simulink model "vardownsampler"  (Simulink 7.3)
settings: Solver=VariableStepDiscrete  StartTime=0.0  StopTime=simTime*SampleTime  RelTol=1e-3
PreLoadFcn:
  | setup_vardownsampler
InitFcn:
  | setup_vardownsampler
values from neighbouring files (symbols this model uses):
  accumOutShift = [1 4 3 2 4]    [setup_vardownsampler.m]    (also in setup_vardownsamplerL8.m = [3 3 2 2 2])
  accumOutWidth = dataWidth + ceil(log2(Rmax))+0    [setup_vardownsampler.m]    (also in setup_vardownsamplerL8.m)
  adderOutShift = 4*ones(1,numRates)    [setup_vardownsampler.m]    (also in setup_vardownsamplerL8.m = 3*ones(1,numRates))
  adderOutWidth = dataWidth + coeffWidth + ceil(log2(L))    [setup_vardownsampler.m]    (also in setup_vardownsamplerL8.m)
  addrWidth = max(1,ceil(log2(Rmax)))    [setup_vardownsampler.m]    (also in setup_vardownsamplerL8.m)
  ChanCount = 16    [setup_vardownsampler.m]    (also in setup_vardownsamplerL8.m = 1)
  ChanCycleCount = ceil(ChanCount/ChanWireCount)    [setup_vardownsampler.m]    (also in setup_vardownsamplerL8.m)
  ChanWireCount = ceil(ChanCount/Period)    [setup_vardownsampler.m]    (also in setup_vardownsamplerL8.m)
  coeffWidth = 16    [setup_vardownsampler.m]    (also in setup_vardownsamplerL8.m)
  dataWidth = 16    [setup_vardownsampler.m]    (also in setup_vardownsamplerL8.m)
  FirAddr = AccumOutScale + 1    (= 4)    [setup_vardownsampler.m]    (also in setup_vardownsamplerL8.m)
  hmatrix = zeros(2*Rmax, L)    [setup_vardownsampler.m]    (also in setup_vardownsamplerL8.m)
  memAddrWidth = max(1,ceil(log2(Nmax)))    [setup_vardownsampler.m]    (also in setup_vardownsamplerL8.m)
  Nmax = Period*Rmax    [setup_vardownsampler.m]    (also in setup_vardownsamplerL8.m)
  Period = floor(ClockRate / SampleRate)    [setup_vardownsampler.m]    (also in setup_vardownsamplerL8.m)
  R = [1 2 5 8 2]    [setup_vardownsampler.m]    (also in setup_vardownsamplerL8.m = [4 5 7 8 9])
  RateWidth = ceil(log2(Rmax))+1    [setup_vardownsampler.m]    (also in setup_vardownsamplerL8.m)
  resetCntWidth = max(1,ceil(log2(Nmax)))    [setup_vardownsampler.m]    (also in setup_vardownsamplerL8.m)
  Rmax = 16    [setup_vardownsampler.m]    (also in setup_vardownsamplerL8.m = 20)
  SampleTime = 1    [setup_vardownsampler.m]    (also in setup_vardownsamplerL8.m)
undefined symbols (not defined in the file or in its folder): AdvDSPBChannelOutDisplay, AdvDSPBDMemDisplay, bank1, bank2, c4, c5, c6, c7, c8, c9, dpoly, dspba_ChannelInVis, dspba_ChannelOutVis, dspba_internal_get_channel_ports, evalAionMaskParam, hmatrix0, hmatrix1, hmatrix2, hmatrix3, latency, primtype, UseDontCare, value
libraries: DSPBAPrim x314, DSPBAModelBus x24, simulink x12, DSPBABase x6
(part 3 of 4)

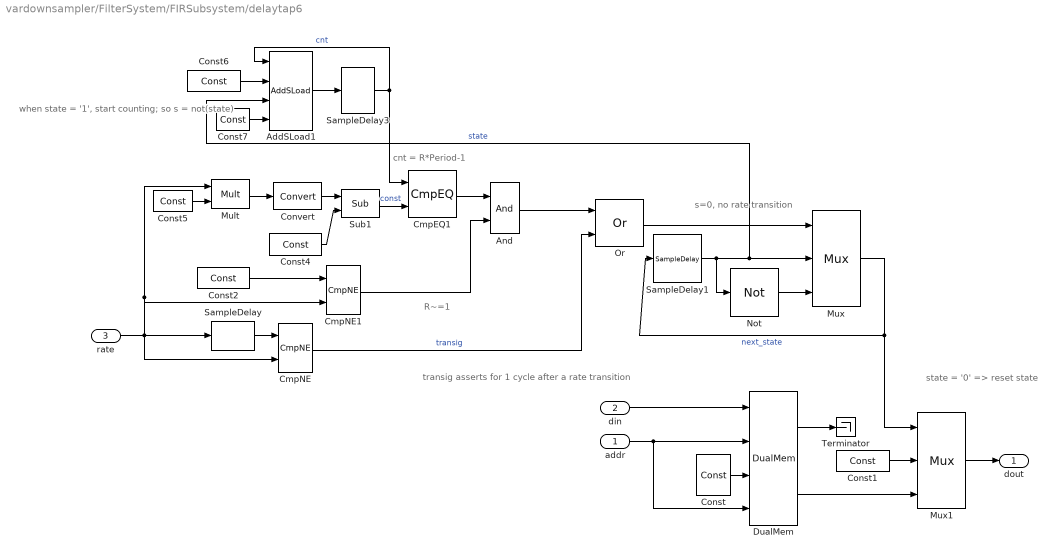
== system vardownsampler/FilterSystem/FIRSubsystem/delaytap6 ==
  note: s=0, no rate transition
  note: transig asserts for 1 cycle after a rate transition
  note: cnt = R*Period-1
  note: when state = '1', start counting;
      | so s = not(state)
  note: state = '0' => reset state
  note: R~=1
  addr : Inport
  din : Inport  Port=2
  rate : Inport  Port=3
  AddSLoad1 : DSPBAPrim/AddSLoad  primtype=addsload  nInputs=4  nOutputs=1  omode=Specify via dialog  otype=uint(resetCntWidth)  scale=1  rndmethod=Unbiased  factor=1  satmethod=Symmetric  shift_vec=[0 1 2 -1]  value=0  inPortNames=['+'; '+'; 's'; 'v']  outPortNames=[' ']  image=dspba_prim.jpg  text=fprintf('+');  style=Optimised  visibilities=8  version=20090407
  And : DSPBAPrim/And  primtype=and  nInputs=2  nOutputs=1  omode=Inherit via internal rule  otype=sfix(16)  scale=2^-15  rndmethod=Unbiased  factor=1  satmethod=Symmetric  shift_vec=[0 1 2 -1]  value=0  inPortNames=[' '; ' '; ' '; ' '; ' '; ' '; ' '; ' '; ' '; ' '; ' '; ' '; ' '; ' '; ' '; ' '; ]  outPortNames=[' ']  image=dspba_prim.jpg  text=fprintf('&');  style=Optimised  visibilities=8+2  version=20090407
  CmpEQ1 : DSPBAPrim/CmpEQ  primtype=cmpeq  nInputs=2  nOutputs=1  omode=boolean  otype=sfix(16)  scale=2^-15  rndmethod=Unbiased  factor=1  satmethod=Symmetric  shift_vec=[0 1 2 -1]  value=0  inPortNames=[' '; ' ';]  outPortNames=[' ']  image=dspba_prim.jpg  text=fprintf('==');  style=Optimised  visibilities=0  version=20090407
  CmpNE : DSPBAPrim/CmpNE  primtype=cmpne  nInputs=2  nOutputs=1  omode=boolean  otype=sfix(16)  scale=2^-15  rndmethod=Unbiased  factor=1  satmethod=Symmetric  shift_vec=[0 1 2 -1]  value=0  inPortNames=[' '; ' ';]  outPortNames=[' ']  image=dspba_prim.jpg  text=fprintf('~=');  style=Optimised  visibilities=0  version=20090407
  CmpNE1 : DSPBAPrim/CmpNE  primtype=cmpne  nInputs=2  nOutputs=1  omode=boolean  otype=sfix(16)  scale=2^-15  rndmethod=Unbiased  factor=1  satmethod=Symmetric  shift_vec=[0 1 2 -1]  value=0  inPortNames=[' '; ' ';]  outPortNames=[' ']  image=dspba_prim.jpg  text=fprintf('~=');  style=Optimised  visibilities=0  version=20090407
  Const : DSPBAPrim/Const  primtype=const  nInputs=0  nOutputs=1  omode=Inherit via internal rule  otype=sfix(16)  scale=2^-15  rndmethod=Unbiased  factor=1  satmethod=Symmetric  shift_vec=[0 1 2 -1]  value=1  inPortNames=['+'; '+';]  outPortNames=[' ']  image=dspba_prim.jpg  text=fprintf('%s', num2str(value));  style=Optimised  visibilities=8 + 1024  version=20090407
  Const1 : DSPBAPrim/Const  primtype=const  nInputs=0  nOutputs=1  omode=Specify via dialog  otype=sfix(dataWidth)  scale=2^(-dataWidth+1)  rndmethod=Unbiased  factor=1  satmethod=Symmetric  shift_vec=[0 1 2 -1]  value=0  inPortNames=['+'; '+';]  outPortNames=[' ']  image=dspba_prim.jpg  text=fprintf('%s', num2str(value));  style=Optimised  visibilities=8 + 1024  version=20090407
  Const2 : DSPBAPrim/Const  primtype=const  nInputs=0  nOutputs=1  omode=Specify via dialog  otype=uint(RateWidth)  scale=1  rndmethod=Unbiased  factor=1  satmethod=Symmetric  shift_vec=[0 1 2 -1]  value=1  inPortNames=['+'; '+';]  outPortNames=[' ']  image=dspba_prim.jpg  text=fprintf('%s', num2str(value));  style=Optimised  visibilities=8 + 1024  version=20090407
  Const4 : DSPBAPrim/Const  primtype=const  nInputs=0  nOutputs=1  omode=Specify via dialog  otype=uint(resetCntWidth)  scale=1  rndmethod=Unbiased  factor=1  satmethod=Symmetric  shift_vec=[0 1 2 -1]  value=1  inPortNames=['+'; '+';]  outPortNames=[' ']  image=dspba_prim.jpg  text=fprintf('%s', num2str(value));  style=Optimised  visibilities=8 + 1024  version=20090407
  Const5 : DSPBAPrim/Const  primtype=const  nInputs=0  nOutputs=1  omode=Specify via dialog  otype=uint(resetCntWidth)  scale=1  rndmethod=Unbiased  factor=1  satmethod=Symmetric  shift_vec=[0 1 2 -1]  value=Period  inPortNames=['+'; '+';]  outPortNames=[' ']  image=dspba_prim.jpg  text=fprintf('%s', num2str(value));  style=Optimised  visibilities=8 + 1024  version=20090407
  Const6 : DSPBAPrim/Const  primtype=const  nInputs=0  nOutputs=1  omode=Specify via dialog  otype=uint(resetCntWidth)  scale=1  rndmethod=Unbiased  factor=1  satmethod=Symmetric  shift_vec=[0 1 2 -1]  value=1  inPortNames=['+'; '+';]  outPortNames=[' ']  image=dspba_prim.jpg  text=fprintf('%s', num2str(value));  style=Optimised  visibilities=8 + 1024  version=20090407
  Const7 : DSPBAPrim/Const  primtype=const  nInputs=0  nOutputs=1  omode=Specify via dialog  otype=uint(resetCntWidth)  scale=1  rndmethod=Unbiased  factor=1  satmethod=Symmetric  shift_vec=[0 1 2 -1]  value=0  inPortNames=['+'; '+';]  outPortNames=[' ']  image=dspba_prim.jpg  text=fprintf('%s', num2str(value));  style=Optimised  visibilities=8 + 1024  version=20090407
  Convert : DSPBAPrim/Convert  primtype=convert  nInputs=1  nOutputs=1  omode=Specify via dialog  otype=uint(resetCntWidth)  scale=1  rndmethod=Truncate  factor=1  satmethod=None  shift_vec=[0 1 2 -1]  value=round([0:255]/17)  inPortNames=[' '; ' ';]  outPortNames=[' '; 'c']  image=dspba_prim.jpg  text=fprintf('convert');  style=Optimised  visibilities=8+64+256  clipdetect=off  version=20090611
  DualMem : DSPBAPrim/DualMem  primtype=dualmem  nInputs=4  nOutputs=2  omode=Inherit via internal rule  otype=sfix(16)  scale=2^-15  rndmethod=Unbiased  factor=1  satmethod=Symmetric  shift_vec=[0 1 2 -1]  value=[zeros(Nmax, 1)]  inPortNames=['d'; 'a'; 'w'; 'a']  outPortNames=['q1'; 'q2']  image=dspba_prim.jpg  text=fprintf('dmem%s',AdvDSPBDMemDisplay(UseDontCare));  style=Optimised  visibilities=8 + 1024  UseDontCare=off  version=20090407
  Mult : DSPBAPrim/Mult  primtype=mult  nInputs=2  nOutputs=1  omode=Inherit via internal rule  otype=sfix(16)  scale=2^-15  rndmethod=Unbiased  factor=1  satmethod=Symmetric  shift_vec=[0 1 2 -1]  value=0  inPortNames=[' '; ' ';]  outPortNames=[' ']  image=dspba_prim.jpg  text=fprintf('X');  style=Optimised  visibilities=8  version=20090407
  Mux : DSPBAPrim/Mux  primtype=mux  nInputs=evalAionMaskParam(gcb,'value',1)+1  nOutputs=1  omode=Inherit via internal rule  otype=sfix(16)  scale=2^-15  rndmethod=Unbiased  factor=1  satmethod=Symmetric  shift_vec=[0 1 2 -1]  value=2  inPortNames=['s'; 'd0'; 'd1'; 'd2'; 'd3'; 'd4'; 'd5'; 'd6'; 'd7'; 'd8'; 'd9';]  outPortNames=[' ']  image=dspba_prim.jpg  text=fprintf('%s', primtype);  style=Optimised  visibilities=1032  version=20090623
  Mux1 : DSPBAPrim/Mux  primtype=mux  nInputs=evalAionMaskParam(gcb,'value',1)+1  nOutputs=1  omode=Inherit via internal rule  otype=sfix(16)  scale=2^-15  rndmethod=Unbiased  factor=1  satmethod=Symmetric  shift_vec=[0 1 2 -1]  value=2  inPortNames=['s'; 'd0'; 'd1'; 'd2'; 'd3'; 'd4'; 'd5'; 'd6'; 'd7'; 'd8'; 'd9';]  outPortNames=[' ']  image=dspba_prim.jpg  text=fprintf('%s', primtype);  style=Optimised  visibilities=1032  version=20090623
  Not : DSPBAPrim/Not  primtype=not  nInputs=1  nOutputs=1  omode=Inherit via internal rule  otype=sfix(16)  scale=2^-15  rndmethod=Unbiased  factor=1  satmethod=Symmetric  shift_vec=[0 1 2 -1]  value=0  inPortNames=[' '; ' ';]  outPortNames=[' ']  image=dspba_prim.jpg  text=fprintf('~');  style=Optimised  visibilities=8  version=20090407
  Or : DSPBAPrim/Or  primtype=or  nInputs=2  nOutputs=1  omode=Inherit via internal rule  otype=sfix(16)  scale=2^-15  rndmethod=Unbiased  factor=1  satmethod=Symmetric  shift_vec=[0 1 2 -1]  value=0  inPortNames=[' '; ' '; ' '; ' '; ' '; ' '; ' '; ' '; ' '; ' '; ' '; ' '; ' '; ' '; ' '; ' '; ]  outPortNames=[' ']  image=dspba_prim.jpg  text=fprintf('|');  style=Optimised  visibilities=8+2  version=20090407
  SampleDelay : DSPBAPrim/SampleDelay  primtype=sampdelay  nInputs=1  nOutputs=1  omode=Inherit via internal rule  otype=sfix(16)  scale=2^-15  rndmethod=Unbiased  factor=1  satmethod=Symmetric  shift_vec=[0 1 2 -1]  value=1  inPortNames=[' '; ' ';]  outPortNames=[' ']  image=dspba_prim.jpg  text=dpoly(1, eye(1,value+1), 'z')  style=Optimised  visibilities=8 + 1024  version=20090407
  SampleDelay1 : DSPBAPrim/SampleDelay  primtype=sampdelay  nInputs=1  nOutputs=1  omode=boolean  otype=sfix(16)  scale=2^-15  rndmethod=Unbiased  factor=1  satmethod=Symmetric  shift_vec=[0 1 2 -1]  value=1  inPortNames=[' '; ' ';]  outPortNames=[' ']  image=dspba_prim.jpg  text=dpoly(1, eye(1,value+1), 'z')  style=Optimised  visibilities=8 + 1024  version=20090407
  SampleDelay3 : DSPBAPrim/SampleDelay  primtype=sampdelay  nInputs=1  nOutputs=1  omode=Inherit via internal rule  otype=uint(memAddrWidth)  scale=1  rndmethod=Unbiased  factor=1  satmethod=Symmetric  shift_vec=[0 1 2 -1]  value=1  inPortNames=[' '; ' ';]  outPortNames=[' ']  image=dspba_prim.jpg  text=dpoly(1, eye(1,value+1), 'z')  style=Optimised  visibilities=8 + 1024  version=20090407
  Sub1 : DSPBAPrim/Sub  primtype=sub  nInputs=2  nOutputs=1  omode=Specify via dialog  otype=uint(memAddrWidth)  scale=1  rndmethod=Unbiased  factor=1  satmethod=Symmetric  shift_vec=[0 1 2 -1]  value=0  inPortNames=['+'; '-';]  outPortNames=[' ']  image=dspba_prim.jpg  text=fprintf('-');  style=Optimised  visibilities=8  version=20090407
  Terminator : Terminator
  dout : Outport  OutDataType=fixdt(1, 16)  OutScaling=2^0
  wires:
  Mux/1 -> SampleDelay1/1, Mux1/1  "next_state"
  SampleDelay/1 -> CmpNE/1
  rate/1 -> SampleDelay/1, CmpNE/2, Mult/1, CmpNE1/2
  CmpNE/1 -> Or/2  "transig"
  Const4/1 -> Sub1/2
  Mult/1 -> Convert/1
  Sub1/1 -> CmpEQ1/2  "const"
  Const5/1 -> Mult/2
  Convert/1 -> Sub1/1
  Const6/1 -> AddSLoad1/2
  AddSLoad1/1 -> SampleDelay3/1
  SampleDelay3/1 -> AddSLoad1/1, CmpEQ1/1  "cnt"
  Const7/1 -> AddSLoad1/4
  Or/1 -> Mux/1
  SampleDelay1/1 -> AddSLoad1/3, Mux/2, Not/1  "state"
  din/1 -> DualMem/1
  addr/1 -> DualMem/2, DualMem/4
  Const/1 -> DualMem/3
  DualMem/1 -> Terminator/1
  Mux1/1 -> dout/1
  Not/1 -> Mux/3
  Const1/1 -> Mux1/2
  DualMem/2 -> Mux1/3
  Const2/1 -> CmpNE1/1
  And/1 -> Or/1
  CmpEQ1/1 -> And/1
  CmpNE1/1 -> And/2

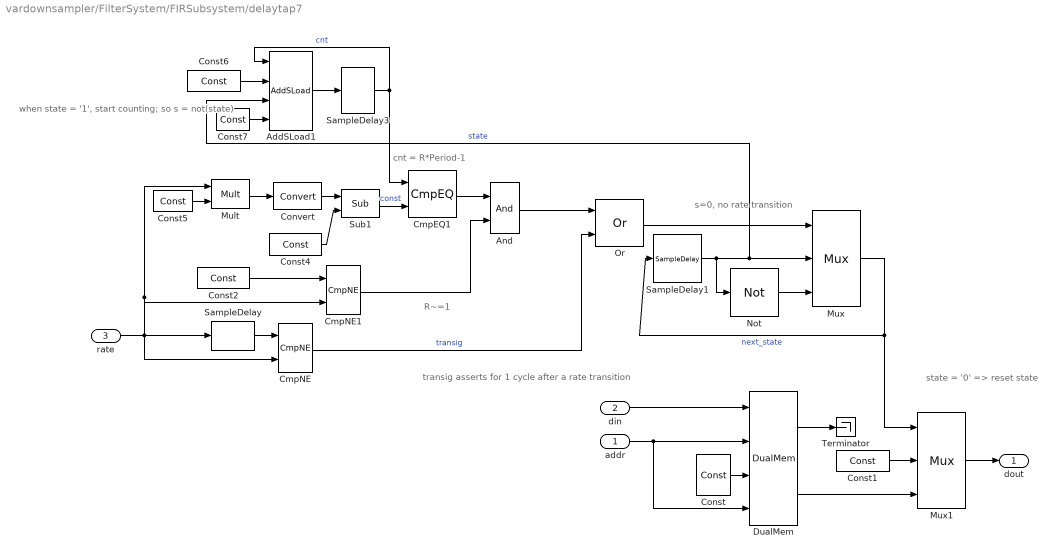
== system vardownsampler/FilterSystem/FIRSubsystem/delaytap7 ==
  note: s=0, no rate transition
  note: transig asserts for 1 cycle after a rate transition
  note: cnt = R*Period-1
  note: when state = '1', start counting;
      | so s = not(state)
  note: state = '0' => reset state
  note: R~=1
  addr : Inport
  din : Inport  Port=2
  rate : Inport  Port=3
  AddSLoad1 : DSPBAPrim/AddSLoad  primtype=addsload  nInputs=4  nOutputs=1  omode=Specify via dialog  otype=uint(resetCntWidth)  scale=1  rndmethod=Unbiased  factor=1  satmethod=Symmetric  shift_vec=[0 1 2 -1]  value=0  inPortNames=['+'; '+'; 's'; 'v']  outPortNames=[' ']  image=dspba_prim.jpg  text=fprintf('+');  style=Optimised  visibilities=8  version=20090407
  And : DSPBAPrim/And  primtype=and  nInputs=2  nOutputs=1  omode=Inherit via internal rule  otype=sfix(16)  scale=2^-15  rndmethod=Unbiased  factor=1  satmethod=Symmetric  shift_vec=[0 1 2 -1]  value=0  inPortNames=[' '; ' '; ' '; ' '; ' '; ' '; ' '; ' '; ' '; ' '; ' '; ' '; ' '; ' '; ' '; ' '; ]  outPortNames=[' ']  image=dspba_prim.jpg  text=fprintf('&');  style=Optimised  visibilities=8+2  version=20090407
  CmpEQ1 : DSPBAPrim/CmpEQ  primtype=cmpeq  nInputs=2  nOutputs=1  omode=boolean  otype=sfix(16)  scale=2^-15  rndmethod=Unbiased  factor=1  satmethod=Symmetric  shift_vec=[0 1 2 -1]  value=0  inPortNames=[' '; ' ';]  outPortNames=[' ']  image=dspba_prim.jpg  text=fprintf('==');  style=Optimised  visibilities=0  version=20090407
  CmpNE : DSPBAPrim/CmpNE  primtype=cmpne  nInputs=2  nOutputs=1  omode=boolean  otype=sfix(16)  scale=2^-15  rndmethod=Unbiased  factor=1  satmethod=Symmetric  shift_vec=[0 1 2 -1]  value=0  inPortNames=[' '; ' ';]  outPortNames=[' ']  image=dspba_prim.jpg  text=fprintf('~=');  style=Optimised  visibilities=0  version=20090407
  CmpNE1 : DSPBAPrim/CmpNE  primtype=cmpne  nInputs=2  nOutputs=1  omode=boolean  otype=sfix(16)  scale=2^-15  rndmethod=Unbiased  factor=1  satmethod=Symmetric  shift_vec=[0 1 2 -1]  value=0  inPortNames=[' '; ' ';]  outPortNames=[' ']  image=dspba_prim.jpg  text=fprintf('~=');  style=Optimised  visibilities=0  version=20090407
  Const : DSPBAPrim/Const  primtype=const  nInputs=0  nOutputs=1  omode=Inherit via internal rule  otype=sfix(16)  scale=2^-15  rndmethod=Unbiased  factor=1  satmethod=Symmetric  shift_vec=[0 1 2 -1]  value=1  inPortNames=['+'; '+';]  outPortNames=[' ']  image=dspba_prim.jpg  text=fprintf('%s', num2str(value));  style=Optimised  visibilities=8 + 1024  version=20090407
  Const1 : DSPBAPrim/Const  primtype=const  nInputs=0  nOutputs=1  omode=Specify via dialog  otype=sfix(dataWidth)  scale=2^(-dataWidth+1)  rndmethod=Unbiased  factor=1  satmethod=Symmetric  shift_vec=[0 1 2 -1]  value=0  inPortNames=['+'; '+';]  outPortNames=[' ']  image=dspba_prim.jpg  text=fprintf('%s', num2str(value));  style=Optimised  visibilities=8 + 1024  version=20090407
  Const2 : DSPBAPrim/Const  primtype=const  nInputs=0  nOutputs=1  omode=Specify via dialog  otype=uint(RateWidth)  scale=1  rndmethod=Unbiased  factor=1  satmethod=Symmetric  shift_vec=[0 1 2 -1]  value=1  inPortNames=['+'; '+';]  outPortNames=[' ']  image=dspba_prim.jpg  text=fprintf('%s', num2str(value));  style=Optimised  visibilities=8 + 1024  version=20090407
  Const4 : DSPBAPrim/Const  primtype=const  nInputs=0  nOutputs=1  omode=Specify via dialog  otype=uint(resetCntWidth)  scale=1  rndmethod=Unbiased  factor=1  satmethod=Symmetric  shift_vec=[0 1 2 -1]  value=1  inPortNames=['+'; '+';]  outPortNames=[' ']  image=dspba_prim.jpg  text=fprintf('%s', num2str(value));  style=Optimised  visibilities=8 + 1024  version=20090407
  Const5 : DSPBAPrim/Const  primtype=const  nInputs=0  nOutputs=1  omode=Specify via dialog  otype=uint(resetCntWidth)  scale=1  rndmethod=Unbiased  factor=1  satmethod=Symmetric  shift_vec=[0 1 2 -1]  value=Period  inPortNames=['+'; '+';]  outPortNames=[' ']  image=dspba_prim.jpg  text=fprintf('%s', num2str(value));  style=Optimised  visibilities=8 + 1024  version=20090407
  Const6 : DSPBAPrim/Const  primtype=const  nInputs=0  nOutputs=1  omode=Specify via dialog  otype=uint(resetCntWidth)  scale=1  rndmethod=Unbiased  factor=1  satmethod=Symmetric  shift_vec=[0 1 2 -1]  value=1  inPortNames=['+'; '+';]  outPortNames=[' ']  image=dspba_prim.jpg  text=fprintf('%s', num2str(value));  style=Optimised  visibilities=8 + 1024  version=20090407
  Const7 : DSPBAPrim/Const  primtype=const  nInputs=0  nOutputs=1  omode=Specify via dialog  otype=uint(resetCntWidth)  scale=1  rndmethod=Unbiased  factor=1  satmethod=Symmetric  shift_vec=[0 1 2 -1]  value=0  inPortNames=['+'; '+';]  outPortNames=[' ']  image=dspba_prim.jpg  text=fprintf('%s', num2str(value));  style=Optimised  visibilities=8 + 1024  version=20090407
  Convert : DSPBAPrim/Convert  primtype=convert  nInputs=1  nOutputs=1  omode=Specify via dialog  otype=uint(resetCntWidth)  scale=1  rndmethod=Truncate  factor=1  satmethod=None  shift_vec=[0 1 2 -1]  value=round([0:255]/17)  inPortNames=[' '; ' ';]  outPortNames=[' '; 'c']  image=dspba_prim.jpg  text=fprintf('convert');  style=Optimised  visibilities=8+64+256  clipdetect=off  version=20090611
  DualMem : DSPBAPrim/DualMem  primtype=dualmem  nInputs=4  nOutputs=2  omode=Inherit via internal rule  otype=sfix(16)  scale=2^-15  rndmethod=Unbiased  factor=1  satmethod=Symmetric  shift_vec=[0 1 2 -1]  value=[zeros(Nmax, 1)]  inPortNames=['d'; 'a'; 'w'; 'a']  outPortNames=['q1'; 'q2']  image=dspba_prim.jpg  text=fprintf('dmem%s',AdvDSPBDMemDisplay(UseDontCare));  style=Optimised  visibilities=8 + 1024  UseDontCare=off  version=20090407
  Mult : DSPBAPrim/Mult  primtype=mult  nInputs=2  nOutputs=1  omode=Inherit via internal rule  otype=sfix(16)  scale=2^-15  rndmethod=Unbiased  factor=1  satmethod=Symmetric  shift_vec=[0 1 2 -1]  value=0  inPortNames=[' '; ' ';]  outPortNames=[' ']  image=dspba_prim.jpg  text=fprintf('X');  style=Optimised  visibilities=8  version=20090407
  Mux : DSPBAPrim/Mux  primtype=mux  nInputs=evalAionMaskParam(gcb,'value',1)+1  nOutputs=1  omode=Inherit via internal rule  otype=sfix(16)  scale=2^-15  rndmethod=Unbiased  factor=1  satmethod=Symmetric  shift_vec=[0 1 2 -1]  value=2  inPortNames=['s'; 'd0'; 'd1'; 'd2'; 'd3'; 'd4'; 'd5'; 'd6'; 'd7'; 'd8'; 'd9';]  outPortNames=[' ']  image=dspba_prim.jpg  text=fprintf('%s', primtype);  style=Optimised  visibilities=1032  version=20090623
  Mux1 : DSPBAPrim/Mux  primtype=mux  nInputs=evalAionMaskParam(gcb,'value',1)+1  nOutputs=1  omode=Inherit via internal rule  otype=sfix(16)  scale=2^-15  rndmethod=Unbiased  factor=1  satmethod=Symmetric  shift_vec=[0 1 2 -1]  value=2  inPortNames=['s'; 'd0'; 'd1'; 'd2'; 'd3'; 'd4'; 'd5'; 'd6'; 'd7'; 'd8'; 'd9';]  outPortNames=[' ']  image=dspba_prim.jpg  text=fprintf('%s', primtype);  style=Optimised  visibilities=1032  version=20090623
  Not : DSPBAPrim/Not  primtype=not  nInputs=1  nOutputs=1  omode=Inherit via internal rule  otype=sfix(16)  scale=2^-15  rndmethod=Unbiased  factor=1  satmethod=Symmetric  shift_vec=[0 1 2 -1]  value=0  inPortNames=[' '; ' ';]  outPortNames=[' ']  image=dspba_prim.jpg  text=fprintf('~');  style=Optimised  visibilities=8  version=20090407
  Or : DSPBAPrim/Or  primtype=or  nInputs=2  nOutputs=1  omode=Inherit via internal rule  otype=sfix(16)  scale=2^-15  rndmethod=Unbiased  factor=1  satmethod=Symmetric  shift_vec=[0 1 2 -1]  value=0  inPortNames=[' '; ' '; ' '; ' '; ' '; ' '; ' '; ' '; ' '; ' '; ' '; ' '; ' '; ' '; ' '; ' '; ]  outPortNames=[' ']  image=dspba_prim.jpg  text=fprintf('|');  style=Optimised  visibilities=8+2  version=20090407
  SampleDelay : DSPBAPrim/SampleDelay  primtype=sampdelay  nInputs=1  nOutputs=1  omode=Inherit via internal rule  otype=sfix(16)  scale=2^-15  rndmethod=Unbiased  factor=1  satmethod=Symmetric  shift_vec=[0 1 2 -1]  value=1  inPortNames=[' '; ' ';]  outPortNames=[' ']  image=dspba_prim.jpg  text=dpoly(1, eye(1,value+1), 'z')  style=Optimised  visibilities=8 + 1024  version=20090407
  SampleDelay1 : DSPBAPrim/SampleDelay  primtype=sampdelay  nInputs=1  nOutputs=1  omode=boolean  otype=sfix(16)  scale=2^-15  rndmethod=Unbiased  factor=1  satmethod=Symmetric  shift_vec=[0 1 2 -1]  value=1  inPortNames=[' '; ' ';]  outPortNames=[' ']  image=dspba_prim.jpg  text=dpoly(1, eye(1,value+1), 'z')  style=Optimised  visibilities=8 + 1024  version=20090407
  SampleDelay3 : DSPBAPrim/SampleDelay  primtype=sampdelay  nInputs=1  nOutputs=1  omode=Inherit via internal rule  otype=uint(memAddrWidth)  scale=1  rndmethod=Unbiased  factor=1  satmethod=Symmetric  shift_vec=[0 1 2 -1]  value=1  inPortNames=[' '; ' ';]  outPortNames=[' ']  image=dspba_prim.jpg  text=dpoly(1, eye(1,value+1), 'z')  style=Optimised  visibilities=8 + 1024  version=20090407
  Sub1 : DSPBAPrim/Sub  primtype=sub  nInputs=2  nOutputs=1  omode=Specify via dialog  otype=uint(memAddrWidth)  scale=1  rndmethod=Unbiased  factor=1  satmethod=Symmetric  shift_vec=[0 1 2 -1]  value=0  inPortNames=['+'; '-';]  outPortNames=[' ']  image=dspba_prim.jpg  text=fprintf('-');  style=Optimised  visibilities=8  version=20090407
  Terminator : Terminator
  dout : Outport  OutDataType=fixdt(1, 16)  OutScaling=2^0
  wires:
  Mux/1 -> SampleDelay1/1, Mux1/1  "next_state"
  SampleDelay/1 -> CmpNE/1
  rate/1 -> SampleDelay/1, CmpNE/2, Mult/1, CmpNE1/2
  CmpNE/1 -> Or/2  "transig"
  Const4/1 -> Sub1/2
  Mult/1 -> Convert/1
  Sub1/1 -> CmpEQ1/2  "const"
  Const5/1 -> Mult/2
  Convert/1 -> Sub1/1
  Const6/1 -> AddSLoad1/2
  AddSLoad1/1 -> SampleDelay3/1
  SampleDelay3/1 -> AddSLoad1/1, CmpEQ1/1  "cnt"
  Const7/1 -> AddSLoad1/4
  Or/1 -> Mux/1
  SampleDelay1/1 -> AddSLoad1/3, Mux/2, Not/1  "state"
  din/1 -> DualMem/1
  addr/1 -> DualMem/2, DualMem/4
  Const/1 -> DualMem/3
  DualMem/1 -> Terminator/1
  Mux1/1 -> dout/1
  Not/1 -> Mux/3
  Const1/1 -> Mux1/2
  DualMem/2 -> Mux1/3
  Const2/1 -> CmpNE1/1
  And/1 -> Or/1
  CmpEQ1/1 -> And/1
  CmpNE1/1 -> And/2

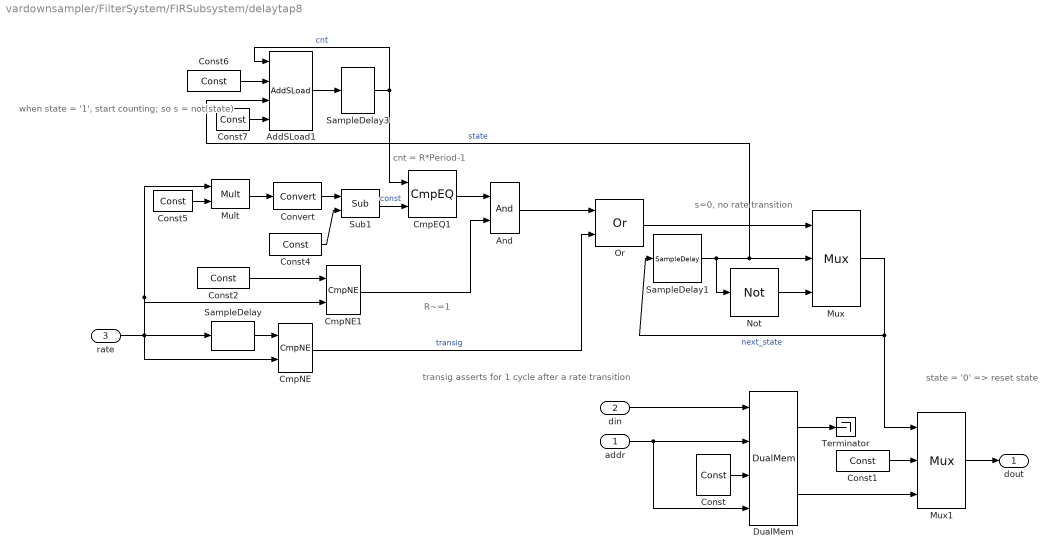
== system vardownsampler/FilterSystem/FIRSubsystem/delaytap8 ==
  note: s=0, no rate transition
  note: transig asserts for 1 cycle after a rate transition
  note: cnt = R*Period-1
  note: when state = '1', start counting;
      | so s = not(state)
  note: state = '0' => reset state
  note: R~=1
  addr : Inport
  din : Inport  Port=2
  rate : Inport  Port=3
  AddSLoad1 : DSPBAPrim/AddSLoad  primtype=addsload  nInputs=4  nOutputs=1  omode=Specify via dialog  otype=uint(resetCntWidth)  scale=1  rndmethod=Unbiased  factor=1  satmethod=Symmetric  shift_vec=[0 1 2 -1]  value=0  inPortNames=['+'; '+'; 's'; 'v']  outPortNames=[' ']  image=dspba_prim.jpg  text=fprintf('+');  style=Optimised  visibilities=8  version=20090407
  And : DSPBAPrim/And  primtype=and  nInputs=2  nOutputs=1  omode=Inherit via internal rule  otype=sfix(16)  scale=2^-15  rndmethod=Unbiased  factor=1  satmethod=Symmetric  shift_vec=[0 1 2 -1]  value=0  inPortNames=[' '; ' '; ' '; ' '; ' '; ' '; ' '; ' '; ' '; ' '; ' '; ' '; ' '; ' '; ' '; ' '; ]  outPortNames=[' ']  image=dspba_prim.jpg  text=fprintf('&');  style=Optimised  visibilities=8+2  version=20090407
  CmpEQ1 : DSPBAPrim/CmpEQ  primtype=cmpeq  nInputs=2  nOutputs=1  omode=boolean  otype=sfix(16)  scale=2^-15  rndmethod=Unbiased  factor=1  satmethod=Symmetric  shift_vec=[0 1 2 -1]  value=0  inPortNames=[' '; ' ';]  outPortNames=[' ']  image=dspba_prim.jpg  text=fprintf('==');  style=Optimised  visibilities=0  version=20090407
  CmpNE : DSPBAPrim/CmpNE  primtype=cmpne  nInputs=2  nOutputs=1  omode=boolean  otype=sfix(16)  scale=2^-15  rndmethod=Unbiased  factor=1  satmethod=Symmetric  shift_vec=[0 1 2 -1]  value=0  inPortNames=[' '; ' ';]  outPortNames=[' ']  image=dspba_prim.jpg  text=fprintf('~=');  style=Optimised  visibilities=0  version=20090407
  CmpNE1 : DSPBAPrim/CmpNE  primtype=cmpne  nInputs=2  nOutputs=1  omode=boolean  otype=sfix(16)  scale=2^-15  rndmethod=Unbiased  factor=1  satmethod=Symmetric  shift_vec=[0 1 2 -1]  value=0  inPortNames=[' '; ' ';]  outPortNames=[' ']  image=dspba_prim.jpg  text=fprintf('~=');  style=Optimised  visibilities=0  version=20090407
  Const : DSPBAPrim/Const  primtype=const  nInputs=0  nOutputs=1  omode=Inherit via internal rule  otype=sfix(16)  scale=2^-15  rndmethod=Unbiased  factor=1  satmethod=Symmetric  shift_vec=[0 1 2 -1]  value=1  inPortNames=['+'; '+';]  outPortNames=[' ']  image=dspba_prim.jpg  text=fprintf('%s', num2str(value));  style=Optimised  visibilities=8 + 1024  version=20090407
  Const1 : DSPBAPrim/Const  primtype=const  nInputs=0  nOutputs=1  omode=Specify via dialog  otype=sfix(dataWidth)  scale=2^(-dataWidth+1)  rndmethod=Unbiased  factor=1  satmethod=Symmetric  shift_vec=[0 1 2 -1]  value=0  inPortNames=['+'; '+';]  outPortNames=[' ']  image=dspba_prim.jpg  text=fprintf('%s', num2str(value));  style=Optimised  visibilities=8 + 1024  version=20090407
  Const2 : DSPBAPrim/Const  primtype=const  nInputs=0  nOutputs=1  omode=Specify via dialog  otype=uint(RateWidth)  scale=1  rndmethod=Unbiased  factor=1  satmethod=Symmetric  shift_vec=[0 1 2 -1]  value=1  inPortNames=['+'; '+';]  outPortNames=[' ']  image=dspba_prim.jpg  text=fprintf('%s', num2str(value));  style=Optimised  visibilities=8 + 1024  version=20090407
  Const4 : DSPBAPrim/Const  primtype=const  nInputs=0  nOutputs=1  omode=Specify via dialog  otype=uint(resetCntWidth)  scale=1  rndmethod=Unbiased  factor=1  satmethod=Symmetric  shift_vec=[0 1 2 -1]  value=1  inPortNames=['+'; '+';]  outPortNames=[' ']  image=dspba_prim.jpg  text=fprintf('%s', num2str(value));  style=Optimised  visibilities=8 + 1024  version=20090407
  Const5 : DSPBAPrim/Const  primtype=const  nInputs=0  nOutputs=1  omode=Specify via dialog  otype=uint(resetCntWidth)  scale=1  rndmethod=Unbiased  factor=1  satmethod=Symmetric  shift_vec=[0 1 2 -1]  value=Period  inPortNames=['+'; '+';]  outPortNames=[' ']  image=dspba_prim.jpg  text=fprintf('%s', num2str(value));  style=Optimised  visibilities=8 + 1024  version=20090407
  Const6 : DSPBAPrim/Const  primtype=const  nInputs=0  nOutputs=1  omode=Specify via dialog  otype=uint(resetCntWidth)  scale=1  rndmethod=Unbiased  factor=1  satmethod=Symmetric  shift_vec=[0 1 2 -1]  value=1  inPortNames=['+'; '+';]  outPortNames=[' ']  image=dspba_prim.jpg  text=fprintf('%s', num2str(value));  style=Optimised  visibilities=8 + 1024  version=20090407
  Const7 : DSPBAPrim/Const  primtype=const  nInputs=0  nOutputs=1  omode=Specify via dialog  otype=uint(resetCntWidth)  scale=1  rndmethod=Unbiased  factor=1  satmethod=Symmetric  shift_vec=[0 1 2 -1]  value=0  inPortNames=['+'; '+';]  outPortNames=[' ']  image=dspba_prim.jpg  text=fprintf('%s', num2str(value));  style=Optimised  visibilities=8 + 1024  version=20090407
  Convert : DSPBAPrim/Convert  primtype=convert  nInputs=1  nOutputs=1  omode=Specify via dialog  otype=uint(resetCntWidth)  scale=1  rndmethod=Truncate  factor=1  satmethod=None  shift_vec=[0 1 2 -1]  value=round([0:255]/17)  inPortNames=[' '; ' ';]  outPortNames=[' '; 'c']  image=dspba_prim.jpg  text=fprintf('convert');  style=Optimised  visibilities=8+64+256  clipdetect=off  version=20090611
  DualMem : DSPBAPrim/DualMem  primtype=dualmem  nInputs=4  nOutputs=2  omode=Inherit via internal rule  otype=sfix(16)  scale=2^-15  rndmethod=Unbiased  factor=1  satmethod=Symmetric  shift_vec=[0 1 2 -1]  value=[zeros(Nmax, 1)]  inPortNames=['d'; 'a'; 'w'; 'a']  outPortNames=['q1'; 'q2']  image=dspba_prim.jpg  text=fprintf('dmem%s',AdvDSPBDMemDisplay(UseDontCare));  style=Optimised  visibilities=8 + 1024  UseDontCare=off  version=20090407
  Mult : DSPBAPrim/Mult  primtype=mult  nInputs=2  nOutputs=1  omode=Inherit via internal rule  otype=sfix(16)  scale=2^-15  rndmethod=Unbiased  factor=1  satmethod=Symmetric  shift_vec=[0 1 2 -1]  value=0  inPortNames=[' '; ' ';]  outPortNames=[' ']  image=dspba_prim.jpg  text=fprintf('X');  style=Optimised  visibilities=8  version=20090407
  Mux : DSPBAPrim/Mux  primtype=mux  nInputs=evalAionMaskParam(gcb,'value',1)+1  nOutputs=1  omode=Inherit via internal rule  otype=sfix(16)  scale=2^-15  rndmethod=Unbiased  factor=1  satmethod=Symmetric  shift_vec=[0 1 2 -1]  value=2  inPortNames=['s'; 'd0'; 'd1'; 'd2'; 'd3'; 'd4'; 'd5'; 'd6'; 'd7'; 'd8'; 'd9';]  outPortNames=[' ']  image=dspba_prim.jpg  text=fprintf('%s', primtype);  style=Optimised  visibilities=1032  version=20090623
  Mux1 : DSPBAPrim/Mux  primtype=mux  nInputs=evalAionMaskParam(gcb,'value',1)+1  nOutputs=1  omode=Inherit via internal rule  otype=sfix(16)  scale=2^-15  rndmethod=Unbiased  factor=1  satmethod=Symmetric  shift_vec=[0 1 2 -1]  value=2  inPortNames=['s'; 'd0'; 'd1'; 'd2'; 'd3'; 'd4'; 'd5'; 'd6'; 'd7'; 'd8'; 'd9';]  outPortNames=[' ']  image=dspba_prim.jpg  text=fprintf('%s', primtype);  style=Optimised  visibilities=1032  version=20090623
  Not : DSPBAPrim/Not  primtype=not  nInputs=1  nOutputs=1  omode=Inherit via internal rule  otype=sfix(16)  scale=2^-15  rndmethod=Unbiased  factor=1  satmethod=Symmetric  shift_vec=[0 1 2 -1]  value=0  inPortNames=[' '; ' ';]  outPortNames=[' ']  image=dspba_prim.jpg  text=fprintf('~');  style=Optimised  visibilities=8  version=20090407
  Or : DSPBAPrim/Or  primtype=or  nInputs=2  nOutputs=1  omode=Inherit via internal rule  otype=sfix(16)  scale=2^-15  rndmethod=Unbiased  factor=1  satmethod=Symmetric  shift_vec=[0 1 2 -1]  value=0  inPortNames=[' '; ' '; ' '; ' '; ' '; ' '; ' '; ' '; ' '; ' '; ' '; ' '; ' '; ' '; ' '; ' '; ]  outPortNames=[' ']  image=dspba_prim.jpg  text=fprintf('|');  style=Optimised  visibilities=8+2  version=20090407
  SampleDelay : DSPBAPrim/SampleDelay  primtype=sampdelay  nInputs=1  nOutputs=1  omode=Inherit via internal rule  otype=sfix(16)  scale=2^-15  rndmethod=Unbiased  factor=1  satmethod=Symmetric  shift_vec=[0 1 2 -1]  value=1  inPortNames=[' '; ' ';]  outPortNames=[' ']  image=dspba_prim.jpg  text=dpoly(1, eye(1,value+1), 'z')  style=Optimised  visibilities=8 + 1024  version=20090407
  SampleDelay1 : DSPBAPrim/SampleDelay  primtype=sampdelay  nInputs=1  nOutputs=1  omode=boolean  otype=sfix(16)  scale=2^-15  rndmethod=Unbiased  factor=1  satmethod=Symmetric  shift_vec=[0 1 2 -1]  value=1  inPortNames=[' '; ' ';]  outPortNames=[' ']  image=dspba_prim.jpg  text=dpoly(1, eye(1,value+1), 'z')  style=Optimised  visibilities=8 + 1024  version=20090407
  SampleDelay3 : DSPBAPrim/SampleDelay  primtype=sampdelay  nInputs=1  nOutputs=1  omode=Inherit via internal rule  otype=uint(memAddrWidth)  scale=1  rndmethod=Unbiased  factor=1  satmethod=Symmetric  shift_vec=[0 1 2 -1]  value=1  inPortNames=[' '; ' ';]  outPortNames=[' ']  image=dspba_prim.jpg  text=dpoly(1, eye(1,value+1), 'z')  style=Optimised  visibilities=8 + 1024  version=20090407
  Sub1 : DSPBAPrim/Sub  primtype=sub  nInputs=2  nOutputs=1  omode=Specify via dialog  otype=uint(memAddrWidth)  scale=1  rndmethod=Unbiased  factor=1  satmethod=Symmetric  shift_vec=[0 1 2 -1]  value=0  inPortNames=['+'; '-';]  outPortNames=[' ']  image=dspba_prim.jpg  text=fprintf('-');  style=Optimised  visibilities=8  version=20090407
  Terminator : Terminator
  dout : Outport  OutDataType=fixdt(1, 16)  OutScaling=2^0
  wires:
  Mux/1 -> SampleDelay1/1, Mux1/1  "next_state"
  SampleDelay/1 -> CmpNE/1
  rate/1 -> SampleDelay/1, CmpNE/2, Mult/1, CmpNE1/2
  CmpNE/1 -> Or/2  "transig"
  Const4/1 -> Sub1/2
  Mult/1 -> Convert/1
  Sub1/1 -> CmpEQ1/2  "const"
  Const5/1 -> Mult/2
  Convert/1 -> Sub1/1
  Const6/1 -> AddSLoad1/2
  AddSLoad1/1 -> SampleDelay3/1
  SampleDelay3/1 -> AddSLoad1/1, CmpEQ1/1  "cnt"
  Const7/1 -> AddSLoad1/4
  Or/1 -> Mux/1
  SampleDelay1/1 -> AddSLoad1/3, Mux/2, Not/1  "state"
  din/1 -> DualMem/1
  addr/1 -> DualMem/2, DualMem/4
  Const/1 -> DualMem/3
  DualMem/1 -> Terminator/1
  Mux1/1 -> dout/1
  Not/1 -> Mux/3
  Const1/1 -> Mux1/2
  DualMem/2 -> Mux1/3
  Const2/1 -> CmpNE1/1
  And/1 -> Or/1
  CmpEQ1/1 -> And/1
  CmpNE1/1 -> And/2

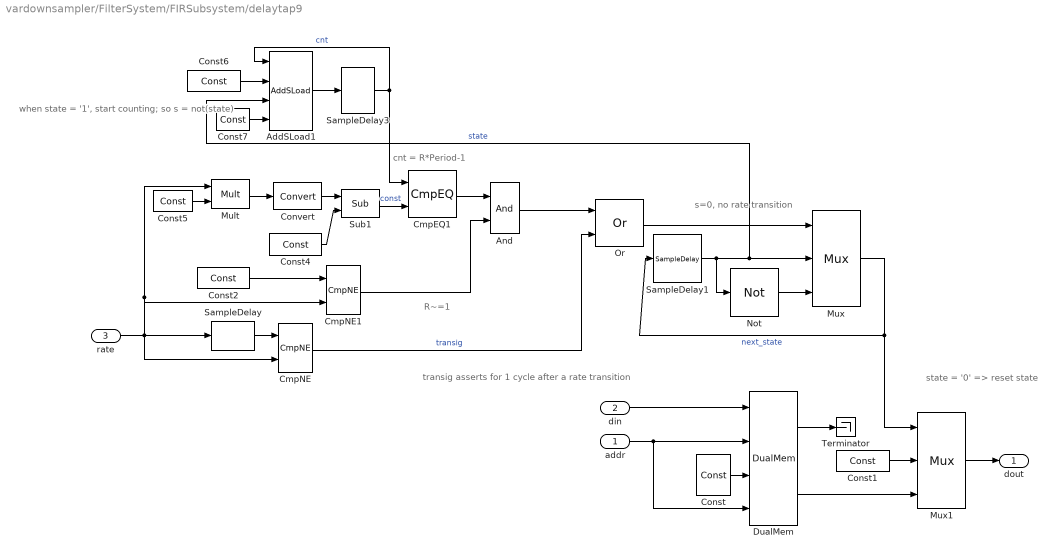
== system vardownsampler/FilterSystem/FIRSubsystem/delaytap9 ==
  note: s=0, no rate transition
  note: transig asserts for 1 cycle after a rate transition
  note: cnt = R*Period-1
  note: when state = '1', start counting;
      | so s = not(state)
  note: state = '0' => reset state
  note: R~=1
  addr : Inport
  din : Inport  Port=2
  rate : Inport  Port=3
  AddSLoad1 : DSPBAPrim/AddSLoad  primtype=addsload  nInputs=4  nOutputs=1  omode=Specify via dialog  otype=uint(resetCntWidth)  scale=1  rndmethod=Unbiased  factor=1  satmethod=Symmetric  shift_vec=[0 1 2 -1]  value=0  inPortNames=['+'; '+'; 's'; 'v']  outPortNames=[' ']  image=dspba_prim.jpg  text=fprintf('+');  style=Optimised  visibilities=8  version=20090407
  And : DSPBAPrim/And  primtype=and  nInputs=2  nOutputs=1  omode=Inherit via internal rule  otype=sfix(16)  scale=2^-15  rndmethod=Unbiased  factor=1  satmethod=Symmetric  shift_vec=[0 1 2 -1]  value=0  inPortNames=[' '; ' '; ' '; ' '; ' '; ' '; ' '; ' '; ' '; ' '; ' '; ' '; ' '; ' '; ' '; ' '; ]  outPortNames=[' ']  image=dspba_prim.jpg  text=fprintf('&');  style=Optimised  visibilities=8+2  version=20090407
  CmpEQ1 : DSPBAPrim/CmpEQ  primtype=cmpeq  nInputs=2  nOutputs=1  omode=boolean  otype=sfix(16)  scale=2^-15  rndmethod=Unbiased  factor=1  satmethod=Symmetric  shift_vec=[0 1 2 -1]  value=0  inPortNames=[' '; ' ';]  outPortNames=[' ']  image=dspba_prim.jpg  text=fprintf('==');  style=Optimised  visibilities=0  version=20090407
  CmpNE : DSPBAPrim/CmpNE  primtype=cmpne  nInputs=2  nOutputs=1  omode=boolean  otype=sfix(16)  scale=2^-15  rndmethod=Unbiased  factor=1  satmethod=Symmetric  shift_vec=[0 1 2 -1]  value=0  inPortNames=[' '; ' ';]  outPortNames=[' ']  image=dspba_prim.jpg  text=fprintf('~=');  style=Optimised  visibilities=0  version=20090407
  CmpNE1 : DSPBAPrim/CmpNE  primtype=cmpne  nInputs=2  nOutputs=1  omode=boolean  otype=sfix(16)  scale=2^-15  rndmethod=Unbiased  factor=1  satmethod=Symmetric  shift_vec=[0 1 2 -1]  value=0  inPortNames=[' '; ' ';]  outPortNames=[' ']  image=dspba_prim.jpg  text=fprintf('~=');  style=Optimised  visibilities=0  version=20090407
  Const : DSPBAPrim/Const  primtype=const  nInputs=0  nOutputs=1  omode=Inherit via internal rule  otype=sfix(16)  scale=2^-15  rndmethod=Unbiased  factor=1  satmethod=Symmetric  shift_vec=[0 1 2 -1]  value=1  inPortNames=['+'; '+';]  outPortNames=[' ']  image=dspba_prim.jpg  text=fprintf('%s', num2str(value));  style=Optimised  visibilities=8 + 1024  version=20090407
  Const1 : DSPBAPrim/Const  primtype=const  nInputs=0  nOutputs=1  omode=Specify via dialog  otype=sfix(dataWidth)  scale=2^(-dataWidth+1)  rndmethod=Unbiased  factor=1  satmethod=Symmetric  shift_vec=[0 1 2 -1]  value=0  inPortNames=['+'; '+';]  outPortNames=[' ']  image=dspba_prim.jpg  text=fprintf('%s', num2str(value));  style=Optimised  visibilities=8 + 1024  version=20090407
  Const2 : DSPBAPrim/Const  primtype=const  nInputs=0  nOutputs=1  omode=Specify via dialog  otype=uint(RateWidth)  scale=1  rndmethod=Unbiased  factor=1  satmethod=Symmetric  shift_vec=[0 1 2 -1]  value=1  inPortNames=['+'; '+';]  outPortNames=[' ']  image=dspba_prim.jpg  text=fprintf('%s', num2str(value));  style=Optimised  visibilities=8 + 1024  version=20090407
  Const4 : DSPBAPrim/Const  primtype=const  nInputs=0  nOutputs=1  omode=Specify via dialog  otype=uint(resetCntWidth)  scale=1  rndmethod=Unbiased  factor=1  satmethod=Symmetric  shift_vec=[0 1 2 -1]  value=1  inPortNames=['+'; '+';]  outPortNames=[' ']  image=dspba_prim.jpg  text=fprintf('%s', num2str(value));  style=Optimised  visibilities=8 + 1024  version=20090407
  Const5 : DSPBAPrim/Const  primtype=const  nInputs=0  nOutputs=1  omode=Specify via dialog  otype=uint(resetCntWidth)  scale=1  rndmethod=Unbiased  factor=1  satmethod=Symmetric  shift_vec=[0 1 2 -1]  value=Period  inPortNames=['+'; '+';]  outPortNames=[' ']  image=dspba_prim.jpg  text=fprintf('%s', num2str(value));  style=Optimised  visibilities=8 + 1024  version=20090407
  Const6 : DSPBAPrim/Const  primtype=const  nInputs=0  nOutputs=1  omode=Specify via dialog  otype=uint(resetCntWidth)  scale=1  rndmethod=Unbiased  factor=1  satmethod=Symmetric  shift_vec=[0 1 2 -1]  value=1  inPortNames=['+'; '+';]  outPortNames=[' ']  image=dspba_prim.jpg  text=fprintf('%s', num2str(value));  style=Optimised  visibilities=8 + 1024  version=20090407
  Const7 : DSPBAPrim/Const  primtype=const  nInputs=0  nOutputs=1  omode=Specify via dialog  otype=uint(resetCntWidth)  scale=1  rndmethod=Unbiased  factor=1  satmethod=Symmetric  shift_vec=[0 1 2 -1]  value=0  inPortNames=['+'; '+';]  outPortNames=[' ']  image=dspba_prim.jpg  text=fprintf('%s', num2str(value));  style=Optimised  visibilities=8 + 1024  version=20090407
  Convert : DSPBAPrim/Convert  primtype=convert  nInputs=1  nOutputs=1  omode=Specify via dialog  otype=uint(resetCntWidth)  scale=1  rndmethod=Truncate  factor=1  satmethod=None  shift_vec=[0 1 2 -1]  value=round([0:255]/17)  inPortNames=[' '; ' ';]  outPortNames=[' '; 'c']  image=dspba_prim.jpg  text=fprintf('convert');  style=Optimised  visibilities=8+64+256  clipdetect=off  version=20090611
  DualMem : DSPBAPrim/DualMem  primtype=dualmem  nInputs=4  nOutputs=2  omode=Inherit via internal rule  otype=sfix(16)  scale=2^-15  rndmethod=Unbiased  factor=1  satmethod=Symmetric  shift_vec=[0 1 2 -1]  value=[zeros(Nmax, 1)]  inPortNames=['d'; 'a'; 'w'; 'a']  outPortNames=['q1'; 'q2']  image=dspba_prim.jpg  text=fprintf('dmem%s',AdvDSPBDMemDisplay(UseDontCare));  style=Optimised  visibilities=8 + 1024  UseDontCare=off  version=20090407
  Mult : DSPBAPrim/Mult  primtype=mult  nInputs=2  nOutputs=1  omode=Inherit via internal rule  otype=sfix(16)  scale=2^-15  rndmethod=Unbiased  factor=1  satmethod=Symmetric  shift_vec=[0 1 2 -1]  value=0  inPortNames=[' '; ' ';]  outPortNames=[' ']  image=dspba_prim.jpg  text=fprintf('X');  style=Optimised  visibilities=8  version=20090407
  Mux : DSPBAPrim/Mux  primtype=mux  nInputs=evalAionMaskParam(gcb,'value',1)+1  nOutputs=1  omode=Inherit via internal rule  otype=sfix(16)  scale=2^-15  rndmethod=Unbiased  factor=1  satmethod=Symmetric  shift_vec=[0 1 2 -1]  value=2  inPortNames=['s'; 'd0'; 'd1'; 'd2'; 'd3'; 'd4'; 'd5'; 'd6'; 'd7'; 'd8'; 'd9';]  outPortNames=[' ']  image=dspba_prim.jpg  text=fprintf('%s', primtype);  style=Optimised  visibilities=1032  version=20090623
  Mux1 : DSPBAPrim/Mux  primtype=mux  nInputs=evalAionMaskParam(gcb,'value',1)+1  nOutputs=1  omode=Inherit via internal rule  otype=sfix(16)  scale=2^-15  rndmethod=Unbiased  factor=1  satmethod=Symmetric  shift_vec=[0 1 2 -1]  value=2  inPortNames=['s'; 'd0'; 'd1'; 'd2'; 'd3'; 'd4'; 'd5'; 'd6'; 'd7'; 'd8'; 'd9';]  outPortNames=[' ']  image=dspba_prim.jpg  text=fprintf('%s', primtype);  style=Optimised  visibilities=1032  version=20090623
  Not : DSPBAPrim/Not  primtype=not  nInputs=1  nOutputs=1  omode=Inherit via internal rule  otype=sfix(16)  scale=2^-15  rndmethod=Unbiased  factor=1  satmethod=Symmetric  shift_vec=[0 1 2 -1]  value=0  inPortNames=[' '; ' ';]  outPortNames=[' ']  image=dspba_prim.jpg  text=fprintf('~');  style=Optimised  visibilities=8  version=20090407
  Or : DSPBAPrim/Or  primtype=or  nInputs=2  nOutputs=1  omode=Inherit via internal rule  otype=sfix(16)  scale=2^-15  rndmethod=Unbiased  factor=1  satmethod=Symmetric  shift_vec=[0 1 2 -1]  value=0  inPortNames=[' '; ' '; ' '; ' '; ' '; ' '; ' '; ' '; ' '; ' '; ' '; ' '; ' '; ' '; ' '; ' '; ]  outPortNames=[' ']  image=dspba_prim.jpg  text=fprintf('|');  style=Optimised  visibilities=8+2  version=20090407
  SampleDelay : DSPBAPrim/SampleDelay  primtype=sampdelay  nInputs=1  nOutputs=1  omode=Inherit via internal rule  otype=sfix(16)  scale=2^-15  rndmethod=Unbiased  factor=1  satmethod=Symmetric  shift_vec=[0 1 2 -1]  value=1  inPortNames=[' '; ' ';]  outPortNames=[' ']  image=dspba_prim.jpg  text=dpoly(1, eye(1,value+1), 'z')  style=Optimised  visibilities=8 + 1024  version=20090407
  SampleDelay1 : DSPBAPrim/SampleDelay  primtype=sampdelay  nInputs=1  nOutputs=1  omode=boolean  otype=sfix(16)  scale=2^-15  rndmethod=Unbiased  factor=1  satmethod=Symmetric  shift_vec=[0 1 2 -1]  value=1  inPortNames=[' '; ' ';]  outPortNames=[' ']  image=dspba_prim.jpg  text=dpoly(1, eye(1,value+1), 'z')  style=Optimised  visibilities=8 + 1024  version=20090407
  SampleDelay3 : DSPBAPrim/SampleDelay  primtype=sampdelay  nInputs=1  nOutputs=1  omode=Inherit via internal rule  otype=uint(memAddrWidth)  scale=1  rndmethod=Unbiased  factor=1  satmethod=Symmetric  shift_vec=[0 1 2 -1]  value=1  inPortNames=[' '; ' ';]  outPortNames=[' ']  image=dspba_prim.jpg  text=dpoly(1, eye(1,value+1), 'z')  style=Optimised  visibilities=8 + 1024  version=20090407
  Sub1 : DSPBAPrim/Sub  primtype=sub  nInputs=2  nOutputs=1  omode=Specify via dialog  otype=uint(memAddrWidth)  scale=1  rndmethod=Unbiased  factor=1  satmethod=Symmetric  shift_vec=[0 1 2 -1]  value=0  inPortNames=['+'; '-';]  outPortNames=[' ']  image=dspba_prim.jpg  text=fprintf('-');  style=Optimised  visibilities=8  version=20090407
  Terminator : Terminator
  dout : Outport  OutDataType=fixdt(1, 16)  OutScaling=2^0
  wires:
  Mux/1 -> SampleDelay1/1, Mux1/1  "next_state"
  SampleDelay/1 -> CmpNE/1
  rate/1 -> SampleDelay/1, CmpNE/2, Mult/1, CmpNE1/2
  CmpNE/1 -> Or/2  "transig"
  Const4/1 -> Sub1/2
  Mult/1 -> Convert/1
  Sub1/1 -> CmpEQ1/2  "const"
  Const5/1 -> Mult/2
  Convert/1 -> Sub1/1
  Const6/1 -> AddSLoad1/2
  AddSLoad1/1 -> SampleDelay3/1
  SampleDelay3/1 -> AddSLoad1/1, CmpEQ1/1  "cnt"
  Const7/1 -> AddSLoad1/4
  Or/1 -> Mux/1
  SampleDelay1/1 -> AddSLoad1/3, Mux/2, Not/1  "state"
  din/1 -> DualMem/1
  addr/1 -> DualMem/2, DualMem/4
  Const/1 -> DualMem/3
  DualMem/1 -> Terminator/1
  Mux1/1 -> dout/1
  Not/1 -> Mux/3
  Const1/1 -> Mux1/2
  DualMem/2 -> Mux1/3
  Const2/1 -> CmpNE1/1
  And/1 -> Or/1
  CmpEQ1/1 -> And/1
  CmpNE1/1 -> And/2

== system vardownsampler/FilterSystem/coefficients_gen/c0 ==
  addr : Inport
  offset : Inport  Port=2
  Const : DSPBAPrim/Const  primtype=const  nInputs=0  nOutputs=1  omode=Specify via dialog  otype=sfix(coeffWidth)  scale=2^-15  rndmethod=Unbiased  factor=1  satmethod=Symmetric  shift_vec=[0 1 2 -1]  value=0  inPortNames=['+'; '+';]  outPortNames=[' ']  image=dspba_prim.jpg  text=fprintf('%s', num2str(value));  style=Optimised  visibilities=8 + 1024  version=20090407
  Const1 : DSPBAPrim/Const  primtype=const  nInputs=0  nOutputs=1  omode=boolean  otype=sfix(16)  scale=2^-15  rndmethod=Unbiased  factor=1  satmethod=Symmetric  shift_vec=[0 1 2 -1]  value=0  inPortNames=['+'; '+';]  outPortNames=[' ']  image=dspba_prim.jpg  text=fprintf('%s', num2str(value));  style=Optimised  visibilities=8 + 1024  version=20090407
  Const2 : DSPBAPrim/Const  primtype=const  nInputs=0  nOutputs=1  omode=Specify via dialog  otype=sfix(coeffWidth)  scale=2^-15  rndmethod=Unbiased  factor=1  satmethod=Symmetric  shift_vec=[0 1 2 -1]  value=0  inPortNames=['+'; '+';]  outPortNames=[' ']  image=dspba_prim.jpg  text=fprintf('%s', num2str(value));  style=Optimised  visibilities=8 + 1024  version=20090407
  Const3 : DSPBAPrim/Const  primtype=const  nInputs=0  nOutputs=1  omode=boolean  otype=sfix(16)  scale=2^-15  rndmethod=Unbiased  factor=1  satmethod=Symmetric  shift_vec=[0 1 2 -1]  value=0  inPortNames=['+'; '+';]  outPortNames=[' ']  image=dspba_prim.jpg  text=fprintf('%s', num2str(value));  style=Optimised  visibilities=8 + 1024  version=20090407
  LUT0 : DSPBAModelBus/SharedMem  mem_addr=FirAddr  mem_rwmode=Read/Write  mem_data=hmatrix(1:Rmax,1)  mem_init=on  mem_desc=hmatrix0 - bank 1  mem_type=sfix(coeffWidth)  mem_scale=2^-(coeffWidth-1)  SampleTime=-1  version=20090407
  LUT1 : DSPBAModelBus/SharedMem  mem_addr=FirAddr + Rmax  mem_rwmode=Read/Write  mem_data=hmatrix(Rmax+1:2*Rmax,1)  mem_init=on  mem_desc=hmatrix0-bank2  mem_type=sfix(coeffWidth)  mem_scale=2^-(coeffWidth-1)  SampleTime=-1  version=20090407
  Mux : DSPBAPrim/Mux  primtype=mux  nInputs=evalAionMaskParam(gcb,'value',1)+1  nOutputs=1  omode=Inherit via internal rule  otype=sfix(16)  scale=2^-15  rndmethod=Unbiased  factor=1  satmethod=Symmetric  shift_vec=[0 1 2 -1]  value=2  inPortNames=['s'; 'd0'; 'd1'; 'd2'; 'd3'; 'd4'; 'd5'; 'd6'; 'd7'; 'd8'; 'd9';]  outPortNames=[' ']  image=dspba_prim.jpg  text=fprintf('%s', primtype);  style=Optimised  visibilities=1032  version=20090623
  c0 : Outport
  wires:
  addr/1 -> LUT0/1, LUT1/1
  Const/1 -> LUT0/2
  Const1/1 -> LUT0/3
  Const2/1 -> LUT1/2
  Const3/1 -> LUT1/3
  offset/1 -> Mux/1
  LUT0/1 -> Mux/2
  LUT1/1 -> Mux/3
  Mux/1 -> c0/1

== system vardownsampler/FilterSystem/coefficients_gen/c1 ==
  addr : Inport
  offset : Inport  Port=2
  Const : DSPBAPrim/Const  primtype=const  nInputs=0  nOutputs=1  omode=Specify via dialog  otype=sfix(coeffWidth)  scale=2^-15  rndmethod=Unbiased  factor=1  satmethod=Symmetric  shift_vec=[0 1 2 -1]  value=0  inPortNames=['+'; '+';]  outPortNames=[' ']  image=dspba_prim.jpg  text=fprintf('%s', num2str(value));  style=Optimised  visibilities=8 + 1024  version=20090407
  Const1 : DSPBAPrim/Const  primtype=const  nInputs=0  nOutputs=1  omode=boolean  otype=sfix(16)  scale=2^-15  rndmethod=Unbiased  factor=1  satmethod=Symmetric  shift_vec=[0 1 2 -1]  value=0  inPortNames=['+'; '+';]  outPortNames=[' ']  image=dspba_prim.jpg  text=fprintf('%s', num2str(value));  style=Optimised  visibilities=8 + 1024  version=20090407
  Const2 : DSPBAPrim/Const  primtype=const  nInputs=0  nOutputs=1  omode=Specify via dialog  otype=sfix(coeffWidth)  scale=2^-15  rndmethod=Unbiased  factor=1  satmethod=Symmetric  shift_vec=[0 1 2 -1]  value=0  inPortNames=['+'; '+';]  outPortNames=[' ']  image=dspba_prim.jpg  text=fprintf('%s', num2str(value));  style=Optimised  visibilities=8 + 1024  version=20090407
  Const3 : DSPBAPrim/Const  primtype=const  nInputs=0  nOutputs=1  omode=boolean  otype=sfix(16)  scale=2^-15  rndmethod=Unbiased  factor=1  satmethod=Symmetric  shift_vec=[0 1 2 -1]  value=0  inPortNames=['+'; '+';]  outPortNames=[' ']  image=dspba_prim.jpg  text=fprintf('%s', num2str(value));  style=Optimised  visibilities=8 + 1024  version=20090407
  LUT0 : DSPBAModelBus/SharedMem  mem_addr=FirAddr+ 2*Rmax  mem_rwmode=Read/Write  mem_data=hmatrix(1:Rmax,2)  mem_init=on  mem_desc=hmatrix1  mem_type=sfix(coeffWidth)  mem_scale=2^-(coeffWidth-1)  SampleTime=-1  version=20090407
  LUT1 : DSPBAModelBus/SharedMem  mem_addr=FirAddr+3*Rmax  mem_rwmode=Read/Write  mem_data=hmatrix(Rmax+1:2*Rmax,2)  mem_init=on  mem_desc=hmatrix1-bank2  mem_type=sfix(coeffWidth)  mem_scale=2^-(coeffWidth-1)  SampleTime=-1  version=20090407
  Mux : DSPBAPrim/Mux  primtype=mux  nInputs=evalAionMaskParam(gcb,'value',1)+1  nOutputs=1  omode=Inherit via internal rule  otype=sfix(16)  scale=2^-15  rndmethod=Unbiased  factor=1  satmethod=Symmetric  shift_vec=[0 1 2 -1]  value=2  inPortNames=['s'; 'd0'; 'd1'; 'd2'; 'd3'; 'd4'; 'd5'; 'd6'; 'd7'; 'd8'; 'd9';]  outPortNames=[' ']  image=dspba_prim.jpg  text=fprintf('%s', primtype);  style=Optimised  visibilities=1032  version=20090623
  c1 : Outport
  wires:
  addr/1 -> LUT0/1, LUT1/1
  Const/1 -> LUT0/2
  Const1/1 -> LUT0/3
  Const2/1 -> LUT1/2
  Const3/1 -> LUT1/3
  LUT0/1 -> Mux/2
  LUT1/1 -> Mux/3
  offset/1 -> Mux/1
  Mux/1 -> c1/1
